simulink subsystem "BatteryMapped"  (R2025a)
settings: Solver=VariableStepAuto  StartTime=0.0  StopTime=10.0  RelTol=1e-3
undefined symbols (not defined in the file): BattAmpHr, BattCurr, BattPwr, BattPwrLoss, BattSoc, BattTemp, BattVolt, PlntBattCp, PlntBattMass, PlntBattNumCellSer
libraries: autolibutils x2, autolibdatasheetbattery x1, autolibpowerinfoutils x1, autolibsharedcommon x1
settings Model: ModifiedByFormat=The MathWorks, Inc.  Creator=The MathWorks, Inc.  LastModifiedBy=The MathWorks, Inc.
settings SolverCC: MaxZcPerStep=1.0
settings OptimizationCC: ReuseModelBlockBuffer=off
settings DebuggingCC: UnconnectedInputMsg=warning  UnconnectedOutputMsg=warning  UnconnectedLineMsg=warning  SubsystemReferenceDiagnosticForUnitTest=warning
settings ModelReferenceCC: EnableRefExpFcnMdlSchedulingChecks=on
settings RTWCC: GPUComputeCapability=3.5  DLArmComputeVersion=19.05  LargeConstantGeneration=WriteOnlyDNNConstantsToDataFiles

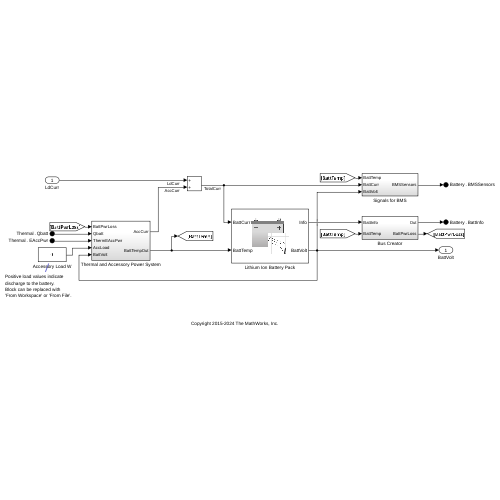
[thumbnail: Simulink's stored preview of the top-level diagram]
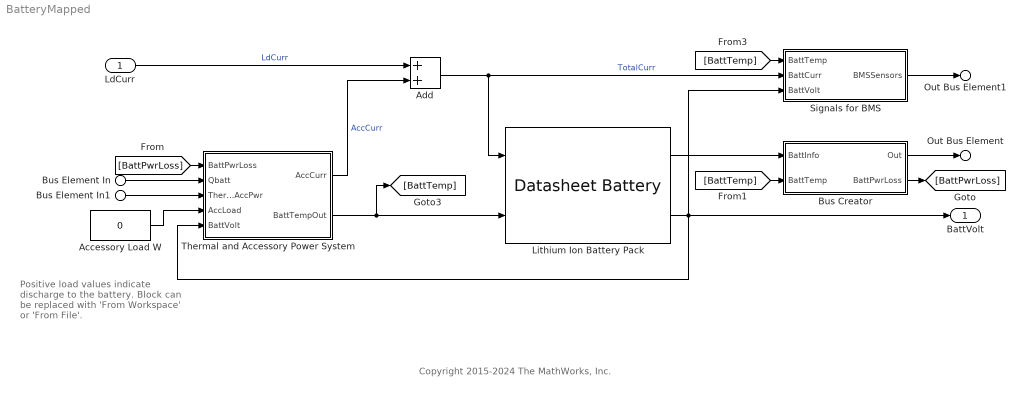
== system BatteryMapped ==
  note: Positive load values indicate
      | discharge to the battery.
      | Block can be replaced with
      | 'From Workspace' or 'From File'.
  note: Copyright 2015-2024 The MathWorks, Inc.
  LdCurr : Inport
  Bus Element In : Inport  Port=2  PortName=Thermal  Element=Qbatt
  Bus Element In1 : Inport  Port=2  PortName=Thermal  Element=EAccPwr
  Accessory Load W : Constant  Value=0
  Add : Sum
  Bus Creator : Subsystem
  Lithium Ion Battery Pack : autolibdatasheetbattery/Datasheet Battery  CapacityCtrl=Parameter  OutputVlt=Filtered  BattChargeMax=PlntBattChrgMax  Em=PlntBattOpenCircVTbl  SOCEmBp=PlntBattVoltSocBpt  RInt=PlntBattIntrnRes'  BattTempBp=PlntBattTempBpt  SOCRintBp=PlntBattSocBpt  Ns=PlntBattNumCellSer  Np=PlntBattNumCellPar  BattCapInit=PlntBattCapInitAh  Tc=PlntBattTimeCnst  Vinit=PlntBattDCDCVinit  RefBlkName='autolibdatasheetbattery/Datasheet Battery'
  Signals for BMS : Subsystem
  Thermal and Accessory Power System : Subsystem
  BattVolt : Outport  VectorParamsAs1DForOutWhenUnconnected=off
  Out Bus Element : Outport  Port=2  PortName=Battery  Element=BattInfo
  Out Bus Element1 : Outport  Port=2  PortName=Battery  Element=BMSSensors
  wires:
  [BattTemp] -> Bus Creator/2(BattTemp)
  Bus Element In1/1 -> Thermal and Accessory Power System/3(ThermEAccPwr)
  Bus Element In/1 -> Thermal and Accessory Power System/2(Qbatt)
  [BattPwrLoss] -> Thermal and Accessory Power System/1(BattPwrLoss)
  Thermal and Accessory Power System/2(BattTempOut) -> Lithium Ion Battery Pack/2, [BattTemp]
  Bus Creator/2(BattPwrLoss) -> [BattPwrLoss]
  Signals for BMS/1(BMSSensors) -> Out Bus Element1/1
  Bus Creator/1(Out) -> Out Bus Element/1
  [BattTemp] -> Signals for BMS/1(BattTemp)
  Lithium Ion Battery Pack/1 -> Bus Creator/1(BattInfo)
  LdCurr/1 -> Add/1  "LdCurr"
  Lithium Ion Battery Pack/2 -> BattVolt/1, Thermal and Accessory Power System/5(BattVolt), Signals for BMS/3(BattVolt)
  Thermal and Accessory Power System/1(AccCurr) -> Add/2  "AccCurr"
  Add/1 -> Lithium Ion Battery Pack/1, Signals for BMS/2(BattCurr)  "TotalCurr"
  Accessory Load W/1 -> Thermal and Accessory Power System/4(AccLoad)

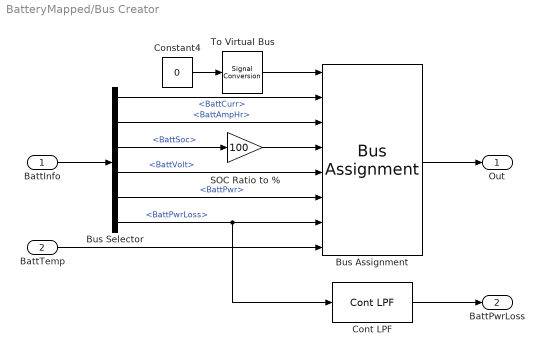
== system BatteryMapped/Bus Creator ==
  BattInfo : Inport
  BattTemp : Inport  Port=2
  Bus Assignment : BusAssignment  AssignedSignals=BattCurr,BattAmpHr,BattSoc,BattVolt,BattPwr,BattPwrLoss,BattTemp
  Bus Selector : BusSelector  OutputSignals=BattCurr,BattAmpHr,BattSoc,BattVolt,BattPwr,BattPwrLoss
  Constant4 : Constant  Value=0  OutDataTypeStr=Bus: BattInfoBUS  SampleTime=Inf
  Cont LPF : autolibutils/Cont LPF  wc=1  AbsoluteTolerance=auto  aMode=6
  SOC Ratio to % : Gain  Gain=100
  To Virtual Bus : SignalConversion  ConversionOutput=Virtual bus  OverrideOpt=off
  Out : Outport
  BattPwrLoss : Outport  Port=2
  wires:
  Cont LPF/1 -> BattPwrLoss/1
  Bus Selector/1 -> Bus Assignment/2  "<BattCurr>"
  SOC Ratio to %/1 -> Bus Assignment/4
  Bus Selector/4 -> Bus Assignment/5  "<BattVolt>"
  To Virtual Bus/1 -> Bus Assignment/1
  Constant4/1 -> To Virtual Bus/1
  BattInfo/1 -> Bus Selector/1
  Bus Selector/3 -> SOC Ratio to %/1  "<BattSoc>"
  Bus Selector/2 -> Bus Assignment/3  "<BattAmpHr>"
  Bus Selector/6 -> Bus Assignment/7, Cont LPF/1  "<BattPwrLoss>"
  Bus Selector/5 -> Bus Assignment/6  "<BattPwr>"
  Bus Assignment/1 -> Out/1
  BattTemp/1 -> Bus Assignment/8

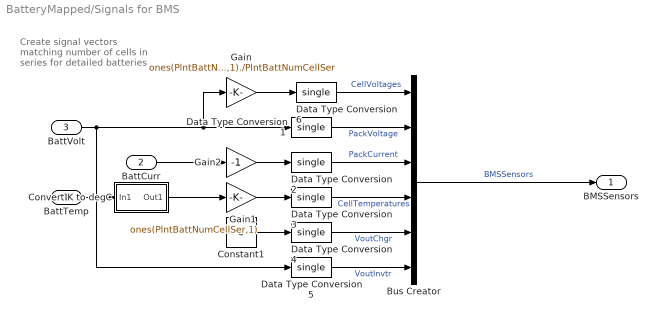
== system BatteryMapped/Signals for BMS ==
  note: Create signal vectors
      | matching number of
      | cells in series for
      | detailed batteries
  BattTemp : Inport
  BattCurr : Inport  Port=2
  BattVolt : Inport  Port=3
  Bus Creator : BusCreator  Inputs=6
  Constant1 : Constant  Value=0
  Convert K to degC : Subsystem
  Data Type Conversion{1..6} (6 alike) : DataTypeConversion  OutDataTypeStr=single  SaturateOnIntegerOverflow=off  RndMeth=Floor
  Gain : Gain  Gain=ones(PlntBattNumCellSer,1)./PlntBattNumCellSer
  Gain1 : Gain  Gain=ones(PlntBattNumCellSer,1)
  Gain2 : Gain  Gain=-1
  BMSSensors : Outport
  wires:
  Bus Creator/1 -> BMSSensors/1  "BMSSensors"
  Data Type Conversion3/1 -> Bus Creator/4  "CellTemperatures"
  Data Type Conversion2/1 -> Bus Creator/3  "PackCurrent"
  Data Type Conversion6/1 -> Bus Creator/1  "CellVoltages"
  Data Type Conversion1/1 -> Bus Creator/2  "PackVoltage"
  Convert K to degC/1(Out1) -> Gain1/1
  Gain2/1 -> Data Type Conversion2/1
  Data Type Conversion5/1 -> Bus Creator/6  "VoutInvtr"
  Gain1/1 -> Data Type Conversion3/1
  Data Type Conversion4/1 -> Bus Creator/5  "VoutChgr"
  BattTemp/1 -> Convert K to degC/1(In1)
  Gain/1 -> Data Type Conversion6/1
  BattVolt/1 -> Data Type Conversion5/1, Gain/1, Data Type Conversion1/1
  Constant1/1 -> Data Type Conversion4/1
  BattCurr/1 -> Gain2/1

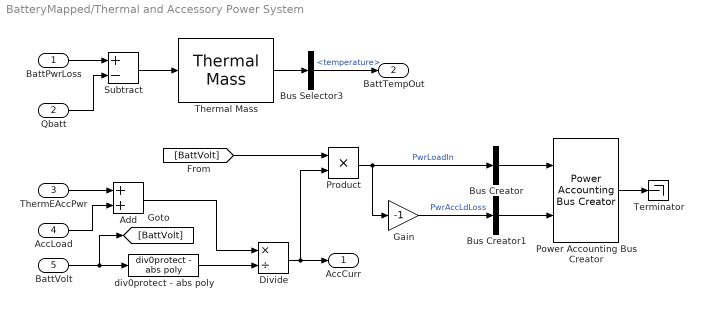
== system BatteryMapped/Thermal and Accessory Power System ==
  BattPwrLoss : Inport
  Qbatt : Inport  Port=2
  ThermEAccPwr : Inport  Port=3
  AccLoad : Inport  Port=4
  BattVolt : Inport  Port=5
  Add : Sum
  Bus Creator : BusCreator  Inputs=1
  Bus Creator1 : BusCreator  Inputs=1
  Bus Selector3 : BusSelector  OutputSignals=temperature
  Divide : Product  Inputs=*/
  Gain : Gain  Gain=-1
  Power Accounting Bus Creator : autolibpowerinfoutils/Power Accounting Bus Creator  AssctBlkSelPopup=Parent  RefBlkName='libraryname/blkname'  PwrTrnsfrdCheckBox=on  PwrNotTrnsfrdCheckBox=on  PwrStoredCheckBox=off  aMode=aMode
  Product : Product
  Subtract : Sum  Inputs=+-
  Terminator : Terminator
  Thermal Mass : autolibsharedcommon/Thermal Mass  MassOrVol=Mass  Mass=PlntBattMass  Volume=10  Rho=997  HeatCp=PlntBattCp*ones(1,2)  HeatBrkPts=PlntBattCpBpt  Tinit=EnvAirTemp  aMode=6
  div0protect - abs poly : autolibutils/div0protect - abs poly  thresh=.001  aMode=6
  AccCurr : Outport
  BattTempOut : Outport  Port=2
  wires:
  Bus Selector3/1 -> BattTempOut/1  "<temperature>"
  Thermal Mass/1 -> Bus Selector3/1
  Qbatt/1 -> Subtract/2
  ThermEAccPwr/1 -> Add/1
  Power Accounting Bus Creator/1 -> Terminator/1
  Bus Creator/1 -> Power Accounting Bus Creator/1
  Bus Creator1/1 -> Power Accounting Bus Creator/2
  Product/1 -> Gain/1, Bus Creator/1  "PwrLoadIn"
  Gain/1 -> Bus Creator1/1  "PwrAccLdLoss"
  Divide/1 -> Product/2, AccCurr/1
  AccLoad/1 -> Add/2
  Add/1 -> Divide/1
  [BattVolt] -> Product/1
  div0protect - abs poly/1 -> Divide/2
  BattVolt/1 -> div0protect - abs poly/1, [BattVolt]
  Subtract/1 -> Thermal Mass/1
  BattPwrLoss/1 -> Subtract/1

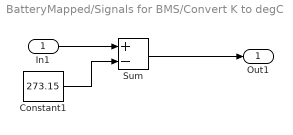
== system BatteryMapped/Signals for BMS/Convert K to degC ==
  In1 : Inport
  Constant1 : Constant  Value=273.15
  Sum : Sum  Inputs=+-
  Out1 : Outport
  wires:
  In1/1 -> Sum/1
  Constant1/1 -> Sum/2
  Sum/1 -> Out1/1
